simulink model "hexa_tilted_quaternion_ANSFT"  (R2023a)
settings: Solver=ode1  StartTime=0.0  StopTime=60  FixedStep=0.01  RelTol=1e-3
undefined symbols (not defined in the file or in its folder): F, Light, MIL
libraries: dspsrcs4 x9, sharedtransform x6, aerolibutil x5, simulink x4, simulink_extras x3, matrix_library x2, sharedutil x2, robotcorelib x1, aerolibwind2 x1, uavutilslib x1
(part 2 of 2)

== matlab function hexa_tilted_quaternion_ANSFT/Reference/Helicoidal Trajectory ==
  data: time input; pose_d output; pose_d_dot output; pose_d_ddot output
function [pose_d, pose_d_dot, pose_d_ddot]= fcn(time)

% pos_z = time / 12;
f = 0.15;
arg = f * (time - 5);
r = 2;

% hover for 5 s | include inclination in roll
% 5 metros al menos

if (time < 5)
    pos_x = 0;
    pos_y = 0;
    % roll = 0;
    pos_z = -0.4 * time;
else
    pos_x = -r + r * cos (arg);
    pos_y = r * sin (arg);
    pos_z = -2;
end

% roll = 0;
% yaw = time * 0;

pose_d = [pos_x;
          pos_y;
          pos_z];
          % roll;
          % 0;
          % yaw];

% pos_z_dot = 1 / 12;

% hover for 5 s
if (time < 5)
    pos_x_dot = 0;
    pos_y_dot = 0;
    pos_z_dot = -0.4;
else
    pos_x_dot = - f * r * sin(arg);
    pos_y_dot = f * r * cos(arg);
    pos_z_dot= 0;
end

% yaw_dot = 0;

pose_d_dot = [pos_x_dot;
              pos_y_dot;
              pos_z_dot];
              % 0;
              % 0;
              % yaw_dot];

pos_z_ddot = 0;
% hover for 5 s
if (time < 5)
    pos_x_ddot = 0;
    pos_y_ddot = 0;
else
    pos_x_ddot = - f * f * r * cos(arg);
    pos_y_ddot = - f * f * r * sin(arg);
end

% yaw_ddot = 0;

pose_d_ddot = [pos_x_ddot;
               pos_y_ddot;
               pos_z_ddot];
               % 0;
               % 0;
               % yaw_ddot];

== matlab function hexa_tilted_quaternion_ANSFT/Reference/Lemniscate Trajectory ==
  data: time input; pose_d output; pose_d_dot output; pose_d_ddot output
function [pose_d, pose_d_dot, pose_d_ddot]= fcn(time)

%% Positions

arg = time / 4;

pos_x = cos(arg) ./ (1 + sin(arg) .* sin(arg));
pos_y = cos(arg) .* sin(arg) ./ (1 + sin(arg) .* sin(arg));
pos_z = sin(arg);

% yaw = time * 0;

pose_d = [pos_x;
          pos_y;
          pos_z];
          % 0;
          % 0;
          % yaw];

%% Velocities

pos_z_dot = 0.25 * cos(arg);
pos_x_dot = - sin(arg)/(4*(sin(arg)^2 + 1)) - (cos(arg)^2*sin(arg))/(2*(sin(arg)^2 + 1)^2);
pos_y_dot = cos(arg)^2/(4*(sin(arg)^2 + 1)) - sin(arg)^2/(4*(sin(arg)^2 + 1)) - (cos(arg)^2*sin(arg)^2)/(2*(sin(arg)^2 + 1)^2);
% yaw_dot = 0;

pose_d_dot = [pos_x_dot;
              pos_y_dot;
              pos_z_dot];
              % 0;
              % 0;
              % yaw_dot];

%% Accelerations

pos_z_ddot = -0.25 * 0.25 * sin(arg);
pos_x_ddot = 0;
pos_y_ddot = 0;
% yaw_ddot = 0;

pose_d_ddot = [pos_x_ddot;
               pos_y_ddot;
               pos_z_ddot];
               % 0;
               % 0;
               % yaw_ddot];

== matlab function hexa_tilted_quaternion_ANSFT/Controller/calculatePWM ==
  data: omega2 input; pwm output
function pwm = fcn(omega2)

pwm = -1.3121e-09 .* omega2 .* omega2 + 0.00208 .* omega2 + 1107.922;
